simulink model "vmc"  (R2020a)
settings: Solver=VariableStepAuto  StartTime=0.0  StopTime=10.0  RelTol=1e-3
undefined symbols (not defined in the file or in its folder): Y1max
settings Model: Creator=solitude  LastModifiedBy=solitude

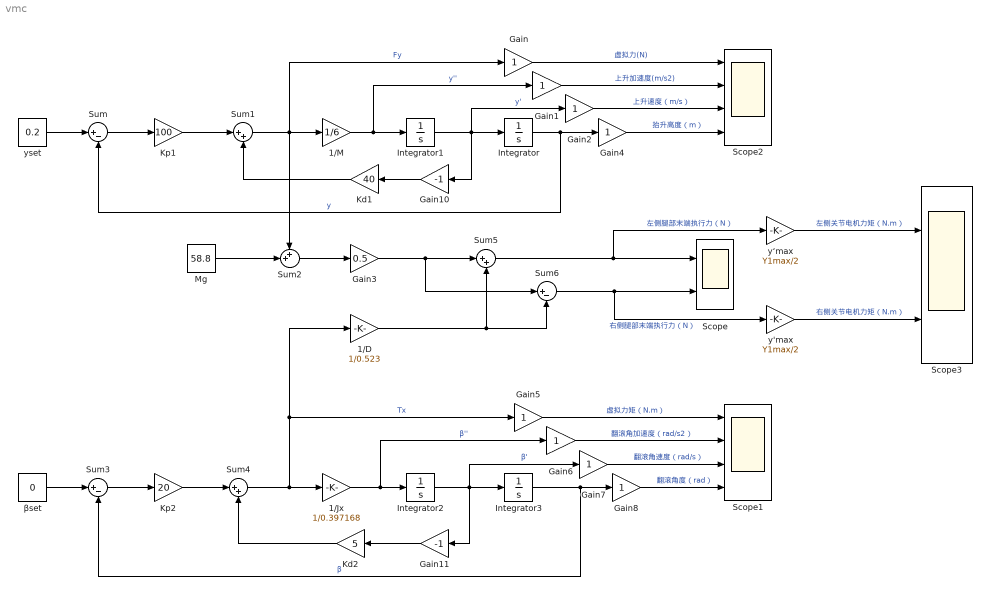
== system vmc ==
  1/D : Gain  Gain=1/0.523
  "1/Jx " : Gain  Gain=1/0.397168
  1/M : Gain  Gain=1/6
  Gain{,1..2,4..8} (8 alike) : Gain
  Gain10 : Gain  Gain=-1
  Gain11 : Gain  Gain=-1
  Gain3 : Gain  Gain=0.5
  Integrator : Integrator
  Integrator1 : Integrator
  Integrator2 : Integrator
  Integrator3 : Integrator  InitialCondition=0.2
  Kd1 : Gain  Gain=40
  Kd2 : Gain  Gain=5
  Kp1 : Gain  Gain=100
  Kp2 : Gain  Gain=20
  Mg : Constant  Value=58.8
  Scope : Scope  NumInputPorts=2
  Scope1 : Scope  NumInputPorts=4
  Scope2 : Scope  NumInputPorts=4
  Scope3 : Scope  NumInputPorts=2
  Sum : Sum  Inputs=|+-
  Sum1 : Sum  Inputs=|++
  Sum2 : Sum  Inputs=++|
  Sum3 : Sum  Inputs=|+-
  Sum4 : Sum  Inputs=|++
  Sum5 : Sum  Inputs=|++
  Sum6 : Sum  Inputs=|+-
  y'max : Gain  Gain=Y1max/2
  yset : Constant  Value=0.2
  y‘max : Gain  Gain=Y1max/2
  βset : Constant  Value=0
  wires:
  yset/1 -> Sum/1
  1/M/1 -> Gain1/1, Integrator1/1  "y''"
  Integrator1/1 -> Gain2/1, Gain10/1, Integrator/1  "y'"
  Integrator/1 -> Gain4/1, Sum/2  "y"
  Sum/1 -> Kp1/1
  Kp1/1 -> Sum1/1
  Kd1/1 -> Sum1/2
  Sum1/1 -> Gain/1, Sum2/1, 1/M/1  "Fy"
  Mg/1 -> Sum2/2
  Sum2/1 -> Gain3/1
  βset/1 -> Sum3/1
  Sum3/1 -> Kp2/1
  Kp2/1 -> Sum4/1
  Sum4/1 -> Gain5/1, 1/D/1, "1/Jx "/1  "Tx"
  "1/Jx "/1 -> Gain6/1, Integrator2/1  "β''"
  Integrator2/1 -> Gain7/1, Integrator3/1, Gain11/1  "β'"
  Integrator3/1 -> Gain8/1, Sum3/2  "β"
  Kd2/1 -> Sum4/2
  Gain3/1 -> Sum6/1, Sum5/1
  Sum5/1 -> y‘max/1, Scope/1  "左侧腿部末端执行力（N）"
  Sum6/1 -> y'max/1, Scope/2  "右侧腿部末端执行力（N）"
  1/D/1 -> Sum6/2, Sum5/2
  y‘max/1 -> Scope3/1  "左侧关节电机力矩（N.m）"
  y'max/1 -> Scope3/2  "右侧关节电机力矩（N.m）"
  Gain10/1 -> Kd1/1
  Gain11/1 -> Kd2/1
  Gain/1 -> Scope2/1  "虚拟力(N)"
  Gain1/1 -> Scope2/2  "上升加速度(m/s2)"
  Gain2/1 -> Scope2/3  "上升速度（m/s）"
  Gain4/1 -> Scope2/4  "抬升高度（m）"
  Gain5/1 -> Scope1/1  "虚拟力矩（N.m）"
  Gain6/1 -> Scope1/2  "翻滚角加速度（rad/s2）"
  Gain7/1 -> Scope1/3  "翻滚角速度（rad/s）"
  Gain8/1 -> Scope1/4  "翻滚角度（rad）"
